simulink model "Motor_Dynamics_Tester"  (Simulink 7.8)
settings: Solver=FixedStepDiscrete  SolverMode=SingleTasking  StartTime=0.0  StopTime=3  FixedStep=0.001  RelTol=1e-3
undefined symbols (not defined in the file or in its folder): DiscIntNeverNeededParam
settings Model: Creator=ft14sl  LastModifiedBy=ft14sl
settings DataIOCC: LimitDataPoints=off  SaveOutput=off  SignalLogging=off  DSMLogging=off  SaveTime=off
settings DebuggingCC: ConsistencyChecking=error  SignalInfNanChecking=error  SignalRangeChecking=error  AlgebraicLoopMsg=error  ArtificialAlgebraicLoopMsg=error  SaveWithDisabledLinksMsg=error  SaveWithParameterizedLinksMsg=error  UnderspecifiedInitializationDetection=Simplified  MergeDetectMultiDrivingBlocksExec=error  BlockPriorityViolationMsg=error  MinStepSizeMsg=error  TimeAdjustmentMsg=warning  SolverPrmCheckMsg=error  InheritedTsInSrcMsg=error  DiscreteInheritContinuousMsg=error  SingleTaskRateTransMsg=error  TasksWithSamePriorityMsg=error  SigSpecEnsureSampleTimeMsg=error  CheckMatrixSingularityMsg=error  IntegerOverflowMsg=error  ParameterUnderflowMsg=error  ParameterPrecisionLossMsg=error  ParameterTunabilityLossMsg=error  FixptConstUnderflowMsg=error  FixptConstOverflowMsg=error  FixptConstPrecisionLossMsg=error  UnderSpecifiedDataTypeMsg=error  UnnecessaryDatatypeConvMsg=warning  VectorMatrixConversionMsg=error  SignalLabelMismatchMsg=error  UnconnectedInputMsg=error  UnconnectedOutputMsg=error  UnconnectedLineMsg=error  SFcnCompatibilityMsg=error  UniqueDataStoreMsg=error  BusObjectLabelMismatch=error  RootOutportRequireBusObject=error  ModelReferenceIOMsg=error  ModelReferenceVersionMismatchMessage=error  ModelReferenceIOMismatchMessage=error  ModelReferenceCSMismatchMessage=error  UnknownTsInhSupMsg=error  ModelReferenceDataLoggingMessage=error  SimStateInterfaceChecksumMismatchMsg=error  StrictBusMsg=ErrorOnBusTreatedAsVector  NonBusSignalsTreatedAsBus=error  SFUnusedDataAndEventsDiag=error  SFUnexpectedBacktrackingDiag=error  SFInvalidInputDataAccessInChartInitDiag=error  SFNoUnconditionalDefaultTransitionDiag=error  SFTransitionOutsideNaturalParentDiag=error  SFUnconditionalTransitionShadowingDiag=error

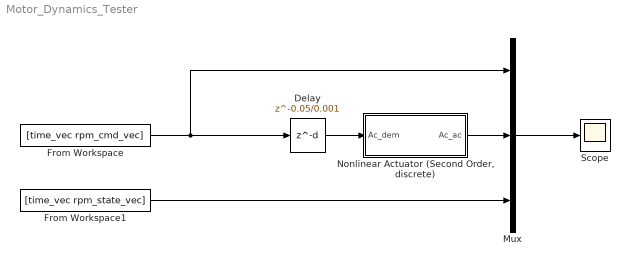
== system Motor_Dynamics_Tester ==
  Delay : Delay  DelayLength=0.05/0.001  InitialCondition=1
  From Workspace : FromWorkspace  VariableName=[time_vec rpm_cmd_vec]  SampleTime=0
  From Workspace1 : FromWorkspace  VariableName=[time_vec rpm_state_vec]  SampleTime=0
  Mux : Mux  Inputs=3
  "Nonlinear Actuator (Second Order, discrete)" : Subsystem  mask(Second Order Nonlinear Actuator ){wn_fin=17, z_fin=0.95, fin_max=inf, fin_min=-inf, fin_maxrate=inf, fin_act_0=[1], offset=0, dt_act=0.001}
      mask prompts: wn_fin "Natural frequency:"; z_fin "Damping ratio:"; fin_max "Maximum deflection:"; fin_min "Minimum deflection:"; fin_maxrate "Maximum rate:"; fin_act_0 "Initial position:"; dt_act "SampleTime"
      mask help: Implement a second-order actuator model with saturation and rate limits.
      mask Help: web(asbhelp);
      mask Display:
      | port_label('input',1,'A_{demand}','texmode','on');
      | port_label('output',1,'A_{actual}','texmode','on');
  Scope : Scope
  wires:
  From Workspace/1 -> Mux/1, Delay/1
  From Workspace1/1 -> Mux/3
  "Nonlinear Actuator (Second Order, discrete)"/1(Ac_ac) -> Mux/2
  Mux/1 -> Scope/1
  Delay/1 -> "Nonlinear Actuator (Second Order, discrete)"/1(Ac_dem)

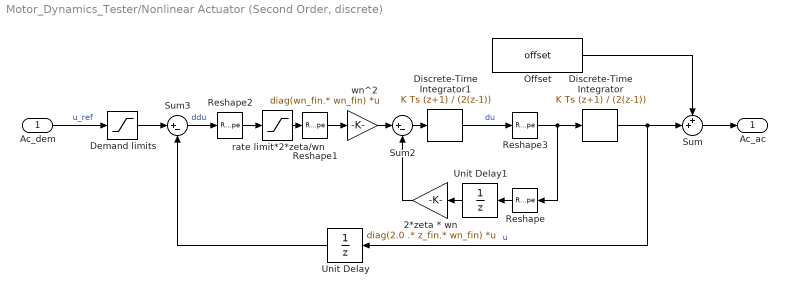
== system Motor_Dynamics_Tester/Nonlinear Actuator (Second Order, discrete) ==
  Ac_dem : Inport
  2*zeta * wn : Gain  Gain=diag(2.0 .* z_fin.* wn_fin)  Multiplication=Matrix(K*u)  SaturateOnIntegerOverflow=on  OutDataTypeStr=Inherit: Same as input  ParamDataTypeStr=Inherit: Same as input
  Demand limits : Saturate  UpperLimit=fin_max  LowerLimit=fin_min
  Discrete-Time Integrator : DiscreteIntegrator  IntegratorMethod=Integration: Trapezoidal  InitialCondition=fin_act_0  SampleTime=dt_act  LimitOutput=on  UpperSaturationLimit=fin_max  LowerSaturationLimit=fin_min  ICPrevOutput=DiscIntNeverNeededParam  ICPrevScaledInput=DiscIntNeverNeededParam
  Discrete-Time Integrator1 : DiscreteIntegrator  IntegratorMethod=Integration: Trapezoidal  SampleTime=dt_act  ICPrevOutput=DiscIntNeverNeededParam  ICPrevScaledInput=DiscIntNeverNeededParam
  Offset : Constant  Value=offset  SampleTime=dt_act
  Reshape : Reshape  OutputDimensionality=Column vector (2-D)
  Reshape1 : Reshape  OutputDimensionality=Column vector (2-D)
  Reshape2 : Reshape
  Reshape3 : Reshape
  Sum : Sum  Inputs=++|
  Sum2 : Sum  Inputs=|+-  SaturateOnIntegerOverflow=on  InputSameDT=on  OutDataTypeStr=Inherit: Same as first input
  Sum3 : Sum  Inputs=|+-  SaturateOnIntegerOverflow=on  InputSameDT=on  OutDataTypeStr=Inherit: Same as first input
  Unit Delay : UnitDelay  X0=fin_act_0  SampleTime=dt_act
  Unit Delay1 : UnitDelay  SampleTime=dt_act
  rate limit*2*zeta/wn : Saturate  UpperLimit=fin_maxrate.*2.*z_fin./wn_fin  LowerLimit=-fin_maxrate.*2.*z_fin./wn_fin
  wn^2 : Gain  Gain=diag(wn_fin.* wn_fin)  Multiplication=Matrix(K*u)  SaturateOnIntegerOverflow=on  OutDataTypeStr=Inherit: Same as input  ParamDataTypeStr=Inherit: Same as input
  Ac_ac : Outport  InitialOutput=0
  wires:
  Unit Delay/1 -> Sum3/2
  Ac_dem/1 -> Demand limits/1  "u_ref"
  Demand limits/1 -> Sum3/1
  rate limit*2*zeta/wn/1 -> Reshape1/1
  Sum3/1 -> Reshape2/1  "ddu"
  2*zeta * wn/1 -> Sum2/2
  Discrete-Time Integrator1/1 -> Reshape3/1  "du"
  Sum2/1 -> Discrete-Time Integrator1/1
  wn^2/1 -> Sum2/1
  Discrete-Time Integrator/1 -> Unit Delay/1, Sum/2  "u"
  Offset/1 -> Sum/1
  Sum/1 -> Ac_ac/1
  Reshape/1 -> Unit Delay1/1
  Reshape1/1 -> wn^2/1
  Reshape2/1 -> rate limit*2*zeta/wn/1
  Reshape3/1 -> Reshape/1, Discrete-Time Integrator/1
  Unit Delay1/1 -> 2*zeta * wn/1
